simulink model "EPS"  (R2020b)
settings: Solver=VariableStepAuto  StartTime=0.0  StopTime=30000  RelTol=1e-3
settings Model: Creator=abelaguiera  LastModifiedBy=abelaguiera

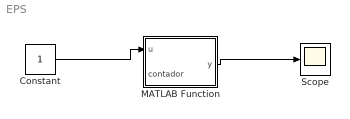
== system EPS ==
  Constant : Constant
  MATLAB Function : MATLAB Function  TreatAsAtomicUnit=on
  Scope : Scope
  wires:
  Constant/1 -> MATLAB Function/1(u)
  MATLAB Function/1(y) -> Scope/1

== matlab function EPS/MATLAB Function ==
  data: u input; y output; contador input
function y = fcn(u, contador)

y = u(contador);
